simulink model "CtrlCmdCalc"  (R2022b)
settings: Solver=FixedStepDiscrete  StartTime=0.0  StopTime=10.0  FixedStep=0.0001  RelTol=1e-3
values from neighbouring files (symbols this model uses):
  Trq_coeff_Arr_Back_60V = 0.0    [MCU_CtrlCmd.sldd]    (also in MCU_CtrlCmd_objects.m = myPackage.Parameter)
  Trq_coeff_Arr_Back_72V = 0.0    [MCU_CtrlCmd.sldd]    (also in MCU_CtrlCmd_objects.m = myPackage.Parameter)
  Trq_coeff_Arr_HSP_60V = 0.0    [MCU_CtrlCmd.sldd]    (also in MCU_CtrlCmd_objects.m = myPackage.Parameter)
  Trq_coeff_Arr_HSP_72V = 0.0    [MCU_CtrlCmd.sldd]    (also in MCU_CtrlCmd_objects.m = myPackage.Parameter)
  TWISTGRIP_HIGH = 3.3    [MCU_CtrlCmd.sldd]
undefined symbols (not defined in the file or in its folder): ANALOG, cNoneMode, cSpeedLoopMode, cTorqueLoopMode, GEAR, MOTORDIR, ParamCfg_CommandSource_u16, ParamCfg_MaxTorque_u16, POWER_ON, PTIME, STANDBY, TWISTGRIP_UP, TWISTGRIP_VTH_HIGH, TWISTGRIP_VTH_UP
libraries: simulink x2
(part 1 of 2)
settings Model: DataDictionary=MCU_CtrlCmd.sldd  Creator=ZYH  LastModifiedBy=ZYH
settings OptimizationCC: DefaultParameterBehavior=Inlined  EnhancedBackFolding=on  PassReuseOutputArgsAs=Individual arguments  ZeroExternalMemoryAtStartup=off  ZeroInternalMemoryAtStartup=off  OptimizeBlockOrder=speed  DifferentSizesBufferReuse=on  OptimizationCustomize=off  EfficientTunableParamExpr=on
settings DebuggingCC: ParameterTunabilityLossMsg=error
settings SFSimCC: MATLABDynamicMemAlloc=off
settings RTWCC: Description=Embedded Coder  SystemTargetFile=ert.tlc  GenCodeOnly=on  TemplateMakefile=ert_default_tmf
settings CodeAppCC: ForceParamTrailComments=on  IgnoreCustomStorageClasses=off  OperatorAnnotations=on  SimulinkDataObjDesc=on  SFDataObjDesc=on  InsertBlockDesc=on
settings ERTTargetCC: TargetLangStandard=C99 (ISO)  GenerateSampleERTMain=on  InlinedParameterPlacement=NonHierarchical  ERTCustomFileTemplate=example_file_process.tlc

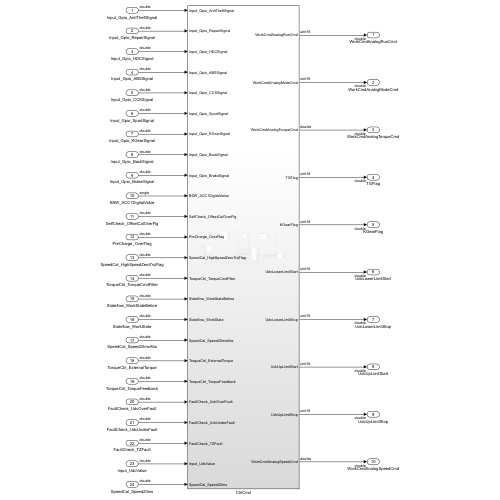
[thumbnail: Simulink's stored preview of the top-level diagram]
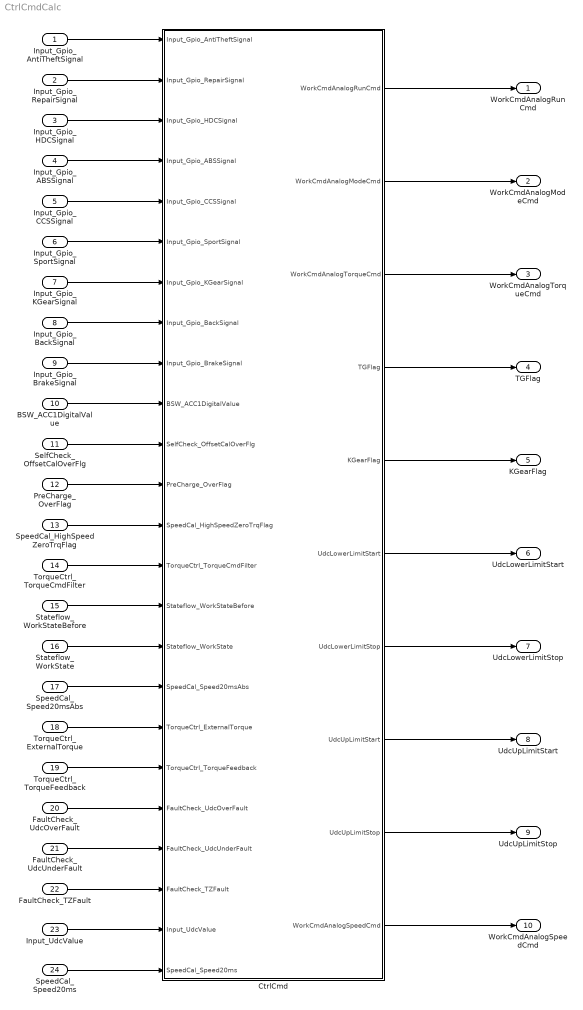
== system CtrlCmdCalc ==
  Input_Gpio_AntiTheftSignal : Inport
  Input_Gpio_RepairSignal : Inport  Port=2
  Input_Gpio_HDCSignal : Inport  Port=3
  Input_Gpio_ABSSignal : Inport  Port=4
  Input_Gpio_CCSSignal : Inport  Port=5
  Input_Gpio_SportSignal : Inport  Port=6
  Input_Gpio_KGearSignal : Inport  Port=7
  Input_Gpio_BackSignal : Inport  Port=8
  Input_Gpio_BrakeSignal : Inport  Port=9
  BSW_ACC1DigitalValue : Inport  Port=10
  SelfCheck_OffsetCalOverFlg : Inport  Port=11
  PreCharge_OverFlag : Inport  Port=12
  SpeedCal_HighSpeedZeroTrqFlag : Inport  Port=13
  TorqueCtrl_TorqueCmdFilter : Inport  Port=14
  Stateflow_WorkStateBefore : Inport  Port=15
  Stateflow_WorkState : Inport  Port=16
  SpeedCal_Speed20msAbs : Inport  Port=17
  TorqueCtrl_ExternalTorque : Inport  Port=18
  TorqueCtrl_TorqueFeedback : Inport  Port=19
  FaultCheck_UdcOverFault : Inport  Port=20
  FaultCheck_UdcUnderFault : Inport  Port=21
  FaultCheck_TZFault : Inport  Port=22
  Input_UdcValue : Inport  Port=23
  SpeedCal_Speed20ms : Inport  Port=24
  CtrlCmd : Subsystem
  WorkCmdAnalogRunCmd : Outport
  WorkCmdAnalogModeCmd : Outport  Port=2
  WorkCmdAnalogTorqueCmd : Outport  Port=3
  TGFlag : Outport  Port=4
  KGearFlag : Outport  Port=5
  UdcLowerLimitStart : Outport  Port=6
  UdcLowerLimitStop : Outport  Port=7
  UdcUpLimitStart : Outport  Port=8
  UdcUpLimitStop : Outport  Port=9
  WorkCmdAnalogSpeedCmd : Outport  Port=10
  wires:
  Input_Gpio_AntiTheftSignal/1 -> CtrlCmd/1(Input_Gpio_AntiTheftSignal)
  Input_Gpio_RepairSignal/1 -> CtrlCmd/2(Input_Gpio_RepairSignal)
  Input_Gpio_HDCSignal/1 -> CtrlCmd/3(Input_Gpio_HDCSignal)
  Input_Gpio_ABSSignal/1 -> CtrlCmd/4(Input_Gpio_ABSSignal)
  Input_Gpio_CCSSignal/1 -> CtrlCmd/5(Input_Gpio_CCSSignal)
  Input_Gpio_SportSignal/1 -> CtrlCmd/6(Input_Gpio_SportSignal)
  Input_Gpio_KGearSignal/1 -> CtrlCmd/7(Input_Gpio_KGearSignal)
  Input_Gpio_BackSignal/1 -> CtrlCmd/8(Input_Gpio_BackSignal)
  Input_Gpio_BrakeSignal/1 -> CtrlCmd/9(Input_Gpio_BrakeSignal)
  BSW_ACC1DigitalValue/1 -> CtrlCmd/10(BSW_ACC1DigitalValue)
  SelfCheck_OffsetCalOverFlg/1 -> CtrlCmd/11(SelfCheck_OffsetCalOverFlg)
  PreCharge_OverFlag/1 -> CtrlCmd/12(PreCharge_OverFlag)
  SpeedCal_HighSpeedZeroTrqFlag/1 -> CtrlCmd/13(SpeedCal_HighSpeedZeroTrqFlag)
  TorqueCtrl_TorqueCmdFilter/1 -> CtrlCmd/14(TorqueCtrl_TorqueCmdFilter)
  Stateflow_WorkStateBefore/1 -> CtrlCmd/15(Stateflow_WorkStateBefore)
  Stateflow_WorkState/1 -> CtrlCmd/16(Stateflow_WorkState)
  SpeedCal_Speed20msAbs/1 -> CtrlCmd/17(SpeedCal_Speed20msAbs)
  TorqueCtrl_ExternalTorque/1 -> CtrlCmd/18(TorqueCtrl_ExternalTorque)
  TorqueCtrl_TorqueFeedback/1 -> CtrlCmd/19(TorqueCtrl_TorqueFeedback)
  FaultCheck_UdcOverFault/1 -> CtrlCmd/20(FaultCheck_UdcOverFault)
  FaultCheck_UdcUnderFault/1 -> CtrlCmd/21(FaultCheck_UdcUnderFault)
  FaultCheck_TZFault/1 -> CtrlCmd/22(FaultCheck_TZFault)
  Input_UdcValue/1 -> CtrlCmd/23(Input_UdcValue)
  SpeedCal_Speed20ms/1 -> CtrlCmd/24(SpeedCal_Speed20ms)
  CtrlCmd/1(WorkCmdAnalogRunCmd) -> WorkCmdAnalogRunCmd/1
  CtrlCmd/2(WorkCmdAnalogModeCmd) -> WorkCmdAnalogModeCmd/1
  CtrlCmd/3(WorkCmdAnalogTorqueCmd) -> WorkCmdAnalogTorqueCmd/1
  CtrlCmd/4(TGFlag) -> TGFlag/1
  CtrlCmd/5(KGearFlag) -> KGearFlag/1
  CtrlCmd/6(UdcLowerLimitStart) -> UdcLowerLimitStart/1
  CtrlCmd/7(UdcLowerLimitStop) -> UdcLowerLimitStop/1
  CtrlCmd/8(UdcUpLimitStart) -> UdcUpLimitStart/1
  CtrlCmd/9(UdcUpLimitStop) -> UdcUpLimitStop/1
  CtrlCmd/10(WorkCmdAnalogSpeedCmd) -> WorkCmdAnalogSpeedCmd/1

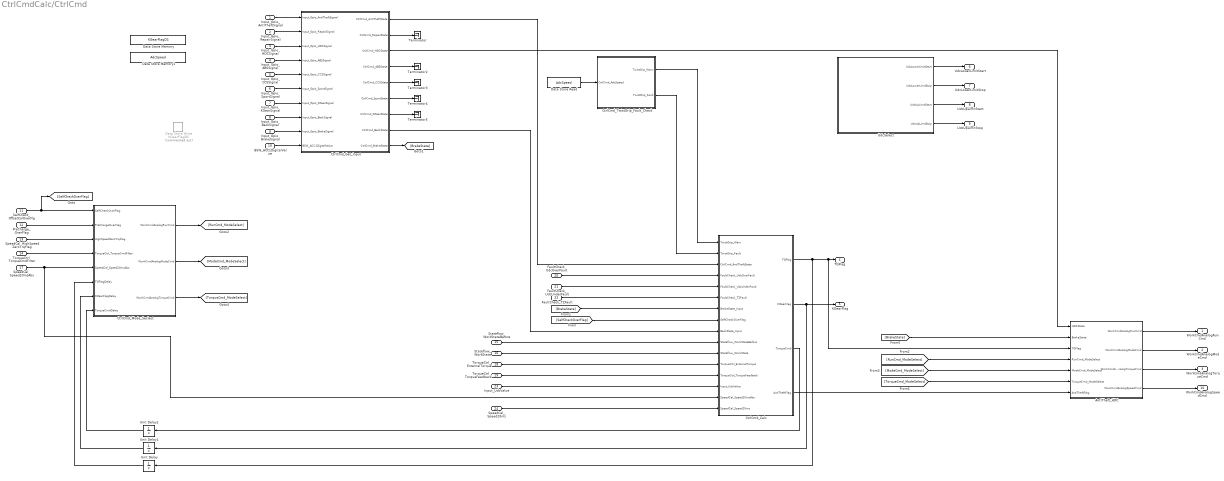
== system CtrlCmdCalc/CtrlCmd ==
  Input_Gpio_AntiTheftSignal : Inport
  Input_Gpio_RepairSignal : Inport  Port=2
  Input_Gpio_HDCSignal : Inport  Port=3
  Input_Gpio_ABSSignal : Inport  Port=4
  Input_Gpio_CCSSignal : Inport  Port=5
  Input_Gpio_SportSignal : Inport  Port=6
  Input_Gpio_KGearSignal : Inport  Port=7
  Input_Gpio_BackSignal : Inport  Port=8
  Input_Gpio_BrakeSignal : Inport  Port=9
  BSW_ACC1DigitalValue : Inport  Port=10
  SelfCheck_OffsetCalOverFlg : Inport  Port=11
  PreCharge_OverFlag : Inport  Port=12
  SpeedCal_HighSpeedZeroTrqFlag : Inport  Port=13
  TorqueCtrl_TorqueCmdFilter : Inport  Port=14
  Stateflow_WorkStateBefore : Inport  Port=15
  Stateflow_WorkState : Inport  Port=16
  SpeedCal_Speed20msAbs : Inport  Port=17
  TorqueCtrl_ExternalTorque : Inport  Port=18
  TorqueCtrl_TorqueFeedback : Inport  Port=19
  FaultCheck_UdcOverFault : Inport  Port=20
  FaultCheck_UdcUnderFault : Inport  Port=21
  FaultCheck_TZFault : Inport  Port=22
  Input_UdcValue : Inport  Port=23
  SpeedCal_Speed20ms : Inport  Port=24
  AntiTheft_HDC : Subsystem
  CtrlCmd_Calc : Subsystem
  CtrlCmd_Get_Input : Subsystem
  CtrlCmd_Mode_Seclect : Subsystem
  CtrlCmd_TwistGrip_Fault_Check : Subsystem
  Data Store Memory : DataStoreMemory  DataStoreName=KGearFlagDS  WriteAfterWriteMsg=warning  InitialValue=3  ShowAdditionalParam=off  OutDataTypeStr=uint16
  Data Store Memory1 : DataStoreMemory  DataStoreName=AdcSpeed  WriteAfterWriteMsg=warning  ShowAdditionalParam=off  OutDataTypeStr=single
  Data Store Read : DataStoreRead  DataStoreName=AdcSpeed  IndexOptions=Index vector (dialog)  Indices=1  OutputSizes=1
  Data Store Write : DataStoreWrite  Commented=on  DataStoreName=KGearFlagDS  IndexOptions=Index vector (dialog)  Indices=1  OutputSizes=1
  Terminator{,2..5} (5 alike) : Terminator
  UdcSelect : Subsystem
  Unit Delay : UnitDelay  SampleTime=-1  HasFrameUpgradeWarning=on
  Unit Delay1 : UnitDelay  SampleTime=-1  HasFrameUpgradeWarning=on
  Unit Delay2 : UnitDelay  SampleTime=-1  HasFrameUpgradeWarning=on
  WorkCmdAnalogRunCmd : Outport
  WorkCmdAnalogModeCmd : Outport  Port=2
  WorkCmdAnalogTorqueCmd : Outport  Port=3
  TGFlag : Outport  Port=4
  KGearFlag : Outport  Port=5
  UdcLowerLimitStart : Outport  Port=6
  UdcLowerLimitStop : Outport  Port=7
  UdcUpLimitStart : Outport  Port=8
  UdcUpLimitStop : Outport  Port=9
  WorkCmdAnalogSpeedCmd : Outport  Port=10
  wires:
  Input_Gpio_AntiTheftSignal/1 -> CtrlCmd_Get_Input/1(Input_Gpio_AntiTheftSignal)
  Input_Gpio_RepairSignal/1 -> CtrlCmd_Get_Input/2(Input_Gpio_RepairSignal)
  Input_Gpio_HDCSignal/1 -> CtrlCmd_Get_Input/3(Input_Gpio_HDCSignal)
  Input_Gpio_ABSSignal/1 -> CtrlCmd_Get_Input/4(Input_Gpio_ABSSignal)
  Input_Gpio_CCSSignal/1 -> CtrlCmd_Get_Input/5(Input_Gpio_CCSSignal)
  Input_Gpio_SportSignal/1 -> CtrlCmd_Get_Input/6(Input_Gpio_SportSignal)
  Input_Gpio_KGearSignal/1 -> CtrlCmd_Get_Input/7(Input_Gpio_KGearSignal)
  Input_Gpio_BackSignal/1 -> CtrlCmd_Get_Input/8(Input_Gpio_BackSignal)
  Input_Gpio_BrakeSignal/1 -> CtrlCmd_Get_Input/9(Input_Gpio_BrakeSignal)
  BSW_ACC1DigitalValue/1 -> CtrlCmd_Get_Input/10(BSW_ACC1DigitalValue)
  SelfCheck_OffsetCalOverFlg/1 -> [SelfCheckOverFlag], CtrlCmd_Mode_Seclect/1(SelfCheckOverFlag)
  Data Store Read/1 -> CtrlCmd_TwistGrip_Fault_Check/1(CtrlCmd_AdcSpeed)
  PreCharge_OverFlag/1 -> CtrlCmd_Mode_Seclect/2(PreChargeOverFlag)
  SpeedCal_HighSpeedZeroTrqFlag/1 -> CtrlCmd_Mode_Seclect/3(HighSpeedZeroTrqFlag)
  TorqueCtrl_TorqueCmdFilter/1 -> CtrlCmd_Mode_Seclect/4(TorqueCtrl_TorqueCmdFilter)
  CtrlCmd_Calc/1(TGFlag) -> AntiTheft_HDC/3(TGFlag), TGFlag/1, Unit Delay/1
  Unit Delay/1 -> CtrlCmd_Mode_Seclect/6(TGFlagDelay)
  CtrlCmd_Calc/2(KGearFlag) -> KGearFlag/1, Unit Delay1/1
  Unit Delay1/1 -> CtrlCmd_Mode_Seclect/7(KGearFlagDelay)
  CtrlCmd_Calc/3(TorqueCmd) -> Unit Delay2/1
  Unit Delay2/1 -> CtrlCmd_Mode_Seclect/8(TorqueCmdDelay)
  SpeedCal_Speed20msAbs/1 -> CtrlCmd_Mode_Seclect/5(SpeedCal_Speed20msAbs), CtrlCmd_Calc/15(SpeedCal_Speed20msAbs)
  Stateflow_WorkStateBefore/1 -> CtrlCmd_Calc/10(Stateflow_WorkStateBefore)
  Stateflow_WorkState/1 -> CtrlCmd_Calc/11(Stateflow_WorkState)
  TorqueCtrl_ExternalTorque/1 -> CtrlCmd_Calc/12(TorqueCtrl_ExternalTorque)
  TorqueCtrl_TorqueFeedback/1 -> CtrlCmd_Calc/13(TorqueCtrl_TorqueFeedback)
  [SelfCheckOverFlag] -> CtrlCmd_Calc/8(SelfCheckOverFlag)
  CtrlCmd_Get_Input/9(CtrlCmd_BrakeState) -> [BrakeState]
  [BrakeState] -> CtrlCmd_Calc/7(BrakeState_Input)
  CtrlCmd_Get_Input/1(CtrlCmd_AntiTheftState) -> CtrlCmd_Calc/3(CtrlCmd_AntiTheftState)
  FaultCheck_TZFault/1 -> CtrlCmd_Calc/6(FaultCheck_TZFault)
  FaultCheck_UdcOverFault/1 -> CtrlCmd_Calc/4(FaultCheck_UdcOverFault)
  FaultCheck_UdcUnderFault/1 -> CtrlCmd_Calc/5(FaultCheck_UdcUnderFault)
  CtrlCmd_TwistGrip_Fault_Check/1(TwistGrip_Warn) -> CtrlCmd_Calc/1(TwistGrip_Warn)
  CtrlCmd_TwistGrip_Fault_Check/2(TwistGrip_Fault) -> CtrlCmd_Calc/2(TwistGrip_Fault)
  CtrlCmd_Get_Input/8(CtrlCmd_BackState) -> CtrlCmd_Calc/9(BackState_Input)
  Input_UdcValue/1 -> CtrlCmd_Calc/14(Input_UdcValue)
  SpeedCal_Speed20ms/1 -> CtrlCmd_Calc/16(SpeedCal_Speed20ms)
  CtrlCmd_Get_Input/2(CtrlCmd_RepairState) -> Terminator/1
  CtrlCmd_Get_Input/4(CtrlCmd_ABSState) -> Terminator2/1
  CtrlCmd_Get_Input/5(CtrlCmd_CCSState) -> Terminator3/1
  CtrlCmd_Get_Input/6(CtrlCmd_SportState) -> Terminator4/1
  CtrlCmd_Get_Input/7(CtrlCmd_KGearState) -> Terminator5/1
  UdcSelect/1(UdcLowerLimitStart) -> UdcLowerLimitStart/1
  UdcSelect/2(UdcLowerLimitStop) -> UdcLowerLimitStop/1
  UdcSelect/3(UdcUpLimitStart) -> UdcUpLimitStart/1
  UdcSelect/4(UdcUpLimitStop) -> UdcUpLimitStop/1
  CtrlCmd_Calc/4(AntiTheftFlag) -> AntiTheft_HDC/7(AntiTheftFlag)
  CtrlCmd_Mode_Seclect/3(WorkCmdAnalogTorqueCmd) -> [TorqueCmd_ModeSelect]
  CtrlCmd_Mode_Seclect/2(WorkCmdAnalogModeCmd) -> [ModeCmd_ModeSelect]
  CtrlCmd_Mode_Seclect/1(WorkCmdAnalogRunCmd) -> [RunCmd_ModeSelect]
  [TorqueCmd_ModeSelect] -> AntiTheft_HDC/6(TorqueCmd_ModeSelect)
  [ModeCmd_ModeSelect] -> AntiTheft_HDC/5(ModeCmd_ModeSelect)
  [RunCmd_ModeSelect] -> AntiTheft_HDC/4(RunCmd_ModeSelect)
  CtrlCmd_Get_Input/3(CtrlCmd_HDCState) -> AntiTheft_HDC/1(HDCState)
  [BrakeState] -> AntiTheft_HDC/2(BrakeState)
  AntiTheft_HDC/1(WorkCmdAnalogRunCmd) -> WorkCmdAnalogRunCmd/1
  AntiTheft_HDC/2(WorkCmdAnalogModeCmd) -> WorkCmdAnalogModeCmd/1
  AntiTheft_HDC/3(WorkCmdAnalogTorqueCmd) -> WorkCmdAnalogTorqueCmd/1
  AntiTheft_HDC/4(WorkCmdAnalogSpeedCmd) -> WorkCmdAnalogSpeedCmd/1

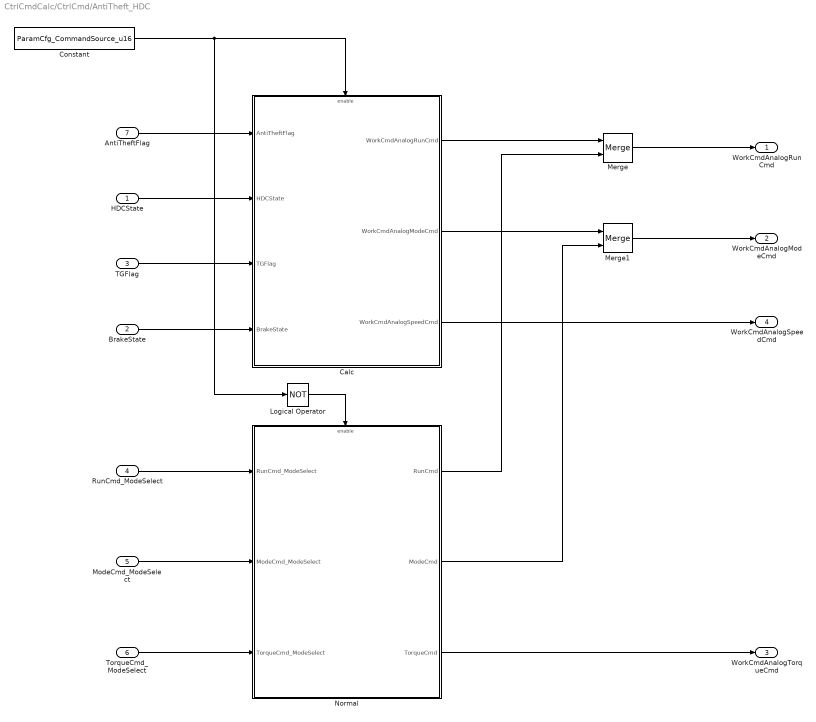
== system CtrlCmdCalc/CtrlCmd/AntiTheft_HDC ==
  HDCState : Inport
  BrakeState : Inport  Port=2
  TGFlag : Inport  Port=3
  RunCmd_ModeSelect : Inport  Port=4
  ModeCmd_ModeSelect : Inport  Port=5
  TorqueCmd_ModeSelect : Inport  Port=6
  AntiTheftFlag : Inport  Port=7
  Calc : Subsystem  TreatAsAtomicUnit=on
  Constant : Constant  Value=ParamCfg_CommandSource_u16
  Logical Operator : Logic  Operator=NOT  AllPortsSameDT=off  OutDataTypeStr=boolean
  Merge : Merge
  Merge1 : Merge
  Normal : Subsystem
  WorkCmdAnalogRunCmd : Outport
  WorkCmdAnalogModeCmd : Outport  Port=2
  WorkCmdAnalogTorqueCmd : Outport  Port=3
  WorkCmdAnalogSpeedCmd : Outport  Port=4
  wires:
  Constant/1 -> Logical Operator/1, Calc/Enable
  AntiTheftFlag/1 -> Calc/1(AntiTheftFlag)
  RunCmd_ModeSelect/1 -> Normal/1(RunCmd_ModeSelect)
  ModeCmd_ModeSelect/1 -> Normal/2(ModeCmd_ModeSelect)
  TorqueCmd_ModeSelect/1 -> Normal/3(TorqueCmd_ModeSelect)
  Logical Operator/1 -> Normal/Enable
  Calc/1(WorkCmdAnalogRunCmd) -> Merge/1
  Merge/1 -> WorkCmdAnalogRunCmd/1
  Calc/2(WorkCmdAnalogModeCmd) -> Merge1/1
  Normal/1(RunCmd) -> Merge/2
  Normal/2(ModeCmd) -> Merge1/2
  Merge1/1 -> WorkCmdAnalogModeCmd/1
  HDCState/1 -> Calc/2(HDCState)
  TGFlag/1 -> Calc/3(TGFlag)
  BrakeState/1 -> Calc/4(BrakeState)
  Calc/3(WorkCmdAnalogSpeedCmd) -> WorkCmdAnalogSpeedCmd/1
  Normal/3(TorqueCmd) -> WorkCmdAnalogTorqueCmd/1

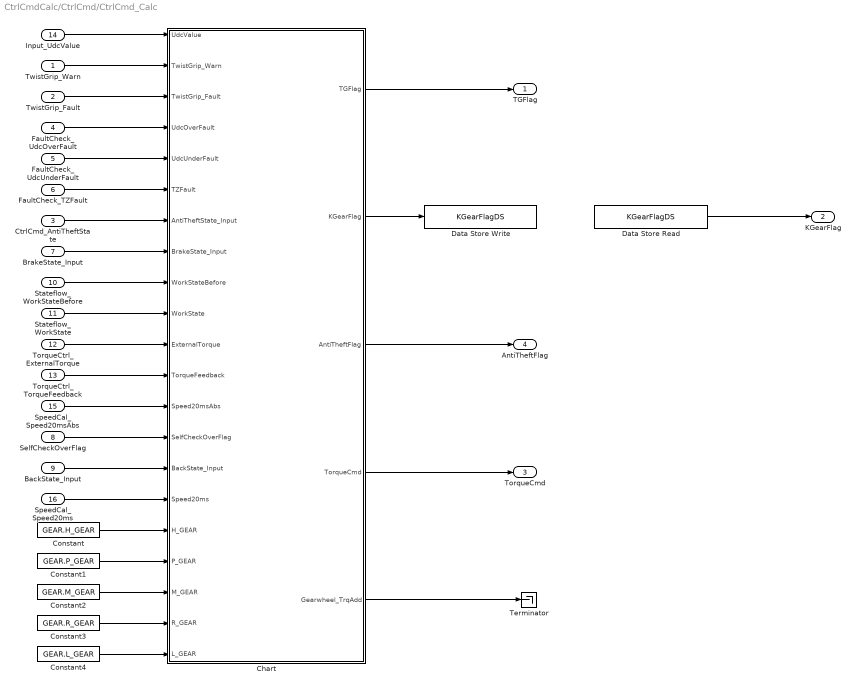
== system CtrlCmdCalc/CtrlCmd/CtrlCmd_Calc ==
  TwistGrip_Warn : Inport
  TwistGrip_Fault : Inport  Port=2
  CtrlCmd_AntiTheftState : Inport  Port=3
  FaultCheck_UdcOverFault : Inport  Port=4
  FaultCheck_UdcUnderFault : Inport  Port=5
  FaultCheck_TZFault : Inport  Port=6
  BrakeState_Input : Inport  Port=7
  SelfCheckOverFlag : Inport  Port=8
  BackState_Input : Inport  Port=9
  Stateflow_WorkStateBefore : Inport  Port=10
  Stateflow_WorkState : Inport  Port=11
  TorqueCtrl_ExternalTorque : Inport  Port=12
  TorqueCtrl_TorqueFeedback : Inport  Port=13
  Input_UdcValue : Inport  Port=14
  SpeedCal_Speed20msAbs : Inport  Port=15
  SpeedCal_Speed20ms : Inport  Port=16
  Chart : Stateflow chart  TreatAsAtomicUnit=on
      settings: PortSchema="{\"entries\":[{\"content\":{\"sides\":[{\"content\":{\"connectorIds\":[\"In1\",\"In3\",\"In2\",\"In5\",\"In4\",\"In6\",\"In7\",\"In8\",\"In9\",\"In10\",\"In11\",\"In12\",\"In13\",\"In15\",\"In20\",\"In21\",\"In14\",\"In16\",\"In17\",\"In18\",\"In19\"]},\"type\":\"ConnectorPlacement.EquallySpacedRectSide\",\"uuid\":\"3ac4e098-dcda-4c80-8391-2c23d040ea90\"},{\"content\":{\"connectorIds\":[\"Out1\",\"Out2\",\"Out3\",\"Out4\",\"Out5\"],\"side\":\"RIGHT\"},\"type\":\"ConnectorPlacement.EquallySpacedRectSide\",\"uuid\":\"2a9563d8-bf95-4ba8-8718-9ed08349656d\"},{\"content\":{\"connectorIds\":[],\"side\":\"TOP\"},\"type\":\"ConnectorPlacement.EquallySpacedRectSide\",\"uuid\":\"a1bb8453-bbab-459c-b3f0-24bc29724271\"}]},\"type\":\"ConnectorPlacement.EquallySpacedConnector\",\"uuid\":\"5f95f66f-474b-4a0c-911a-4da2c08bb750\"}],\"packageUris\":[\"http://schema.mathworks.com/mf0/Connector/R2020b\"],\"version\":\"1.0\"}"
  Constant : Constant  Value=GEAR.H_GEAR
  Constant1 : Constant  Value=GEAR.P_GEAR
  Constant2 : Constant  Value=GEAR.M_GEAR
  Constant3 : Constant  Value=GEAR.R_GEAR
  Constant4 : Constant  Value=GEAR.L_GEAR
  Data Store Read : DataStoreRead  DataStoreName=KGearFlagDS  IndexOptions=Index vector (dialog)  Indices=1  OutputSizes=1
  Data Store Write : DataStoreWrite  DataStoreName=KGearFlagDS  IndexOptions=Index vector (dialog)  Indices=1  OutputSizes=1
  Terminator : Terminator
  TGFlag : Outport
  KGearFlag : Outport  Port=2
  TorqueCmd : Outport  Port=3
  AntiTheftFlag : Outport  Port=4
  wires:
  Stateflow_WorkStateBefore/1 -> Chart/9(WorkStateBefore)
  Stateflow_WorkState/1 -> Chart/10(WorkState)
  TorqueCtrl_ExternalTorque/1 -> Chart/11(ExternalTorque)
  TorqueCtrl_TorqueFeedback/1 -> Chart/12(TorqueFeedback)
  SpeedCal_Speed20msAbs/1 -> Chart/13(Speed20msAbs)
  Chart/2(KGearFlag) -> Data Store Write/1
  Constant/1 -> Chart/14(H_GEAR)
  SelfCheckOverFlag/1 -> Chart/15(SelfCheckOverFlag)
  Constant1/1 -> Chart/16(P_GEAR)
  BrakeState_Input/1 -> Chart/8(BrakeState_Input)
  Constant2/1 -> Chart/17(M_GEAR)
  Data Store Read/1 -> KGearFlag/1
  Chart/1(TGFlag) -> TGFlag/1
  Constant3/1 -> Chart/18(R_GEAR)
  CtrlCmd_AntiTheftState/1 -> Chart/7(AntiTheftState_Input)
  Chart/3(AntiTheftFlag) -> AntiTheftFlag/1
  TwistGrip_Warn/1 -> Chart/3(TwistGrip_Warn)
  TwistGrip_Fault/1 -> Chart/2(TwistGrip_Fault)
  FaultCheck_UdcOverFault/1 -> Chart/5(UdcOverFault)
  FaultCheck_UdcUnderFault/1 -> Chart/4(UdcUnderFault)
  FaultCheck_TZFault/1 -> Chart/6(TZFault)
  Constant4/1 -> Chart/19(L_GEAR)
  BackState_Input/1 -> Chart/20(BackState_Input)
  Chart/4(TorqueCmd) -> TorqueCmd/1
  Input_UdcValue/1 -> Chart/1(UdcValue)
  Chart/5(Gearwheel_TrqAdd) -> Terminator/1
  SpeedCal_Speed20ms/1 -> Chart/21(Speed20ms)

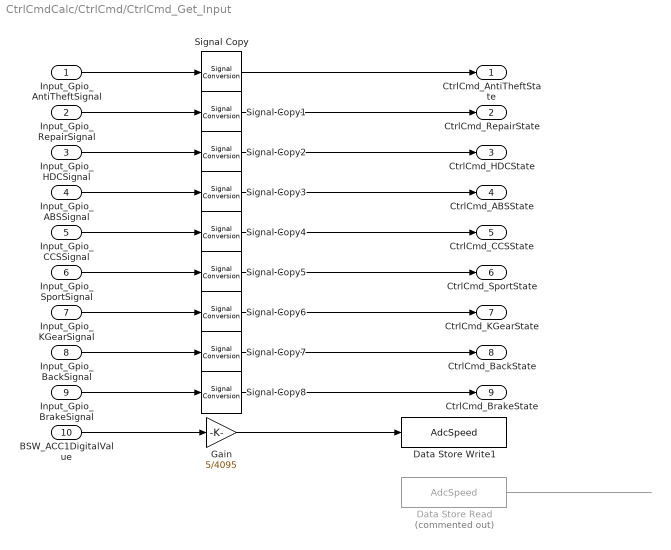
== system CtrlCmdCalc/CtrlCmd/CtrlCmd_Get_Input ==
  Input_Gpio_AntiTheftSignal : Inport
  Input_Gpio_RepairSignal : Inport  Port=2
  Input_Gpio_HDCSignal : Inport  Port=3
  Input_Gpio_ABSSignal : Inport  Port=4
  Input_Gpio_CCSSignal : Inport  Port=5
  Input_Gpio_SportSignal : Inport  Port=6
  Input_Gpio_KGearSignal : Inport  Port=7
  Input_Gpio_BackSignal : Inport  Port=8
  Input_Gpio_BrakeSignal : Inport  Port=9
  BSW_ACC1DigitalValue : Inport  Port=10
  Data Store Read : DataStoreRead  Commented=on  DataStoreName=AdcSpeed  IndexOptions=Index vector (dialog)  Indices=1  OutputSizes=1
  Data Store Write1 : DataStoreWrite  DataStoreName=AdcSpeed  IndexOptions=Index vector (dialog)  Indices=1  OutputSizes=1
  Gain : Gain  Gain=5/4095  ParamDataTypeStr=single  OutDataTypeStr=single
      settings: AttributesFormatString=%<Gain>
  Signal Copy{,1..8} (9 alike) : SignalConversion  OverrideOpt=off
  CtrlCmd_AntiTheftState : Outport
  CtrlCmd_RepairState : Outport  Port=2
  CtrlCmd_HDCState : Outport  Port=3
  CtrlCmd_ABSState : Outport  Port=4
  CtrlCmd_CCSState : Outport  Port=5
  CtrlCmd_SportState : Outport  Port=6
  CtrlCmd_KGearState : Outport  Port=7
  CtrlCmd_BackState : Outport  Port=8
  CtrlCmd_BrakeState : Outport  Port=9
  wires:
  Input_Gpio_AntiTheftSignal/1 -> Signal Copy/1
  Input_Gpio_RepairSignal/1 -> Signal Copy1/1
  Input_Gpio_HDCSignal/1 -> Signal Copy2/1
  Input_Gpio_ABSSignal/1 -> Signal Copy3/1
  Input_Gpio_CCSSignal/1 -> Signal Copy4/1
  Input_Gpio_SportSignal/1 -> Signal Copy5/1
  Input_Gpio_KGearSignal/1 -> Signal Copy6/1
  Input_Gpio_BackSignal/1 -> Signal Copy7/1
  Input_Gpio_BrakeSignal/1 -> Signal Copy8/1
  BSW_ACC1DigitalValue/1 -> Gain/1
  Gain/1 -> Data Store Write1/1
  Signal Copy/1 -> CtrlCmd_AntiTheftState/1
  Signal Copy1/1 -> CtrlCmd_RepairState/1
  Signal Copy8/1 -> CtrlCmd_BrakeState/1
  Signal Copy7/1 -> CtrlCmd_BackState/1
  Signal Copy6/1 -> CtrlCmd_KGearState/1
  Signal Copy5/1 -> CtrlCmd_SportState/1
  Signal Copy4/1 -> CtrlCmd_CCSState/1
  Signal Copy3/1 -> CtrlCmd_ABSState/1
  Signal Copy2/1 -> CtrlCmd_HDCState/1
  Data Store Read/1 -> ?

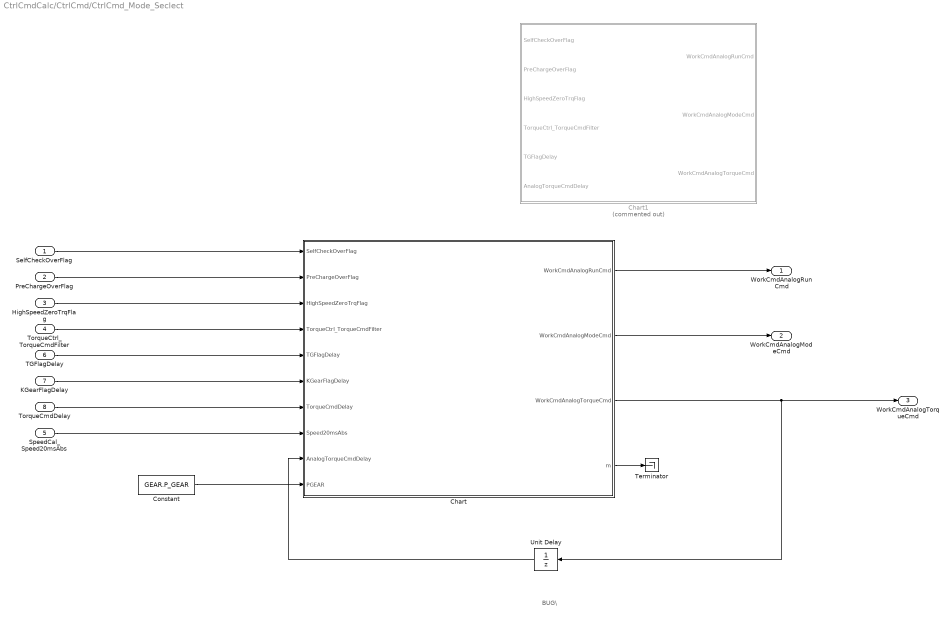
== system CtrlCmdCalc/CtrlCmd/CtrlCmd_Mode_Seclect ==
  note: BUG\
  SelfCheckOverFlag : Inport
  PreChargeOverFlag : Inport  Port=2
  HighSpeedZeroTrqFlag : Inport  Port=3
  TorqueCtrl_TorqueCmdFilter : Inport  Port=4
  SpeedCal_Speed20msAbs : Inport  Port=5
  TGFlagDelay : Inport  Port=6
  KGearFlagDelay : Inport  Port=7
  TorqueCmdDelay : Inport  Port=8
  Chart : Stateflow chart  TreatAsAtomicUnit=on
      settings: PortSchema="{\"entries\":[{\"content\":{\"sides\":[{\"content\":{\"connectorIds\":[\"In1\",\"In2\",\"In3\",\"In4\",\"In5\",\"In9\",\"In7\",\"In8\",\"In6\",\"In10\"]},\"type\":\"ConnectorPlacement.EquallySpacedRectSide\",\"uuid\":\"b2d776f0-2615-48a9-a6c0-c843049782f9\"},{\"content\":{\"connectorIds\":[\"Out1\",\"Out2\",\"Out3\",\"Out4\"],\"side\":\"RIGHT\"},\"type\":\"ConnectorPlacement.EquallySpacedRectSide\",\"uuid\":\"8bd2f04f-8b65-482d-924a-cc36ec8f1c20\"},{\"content\":{\"connectorIds\":[],\"side\":\"TOP\"},\"type\":\"ConnectorPlacement.EquallySpacedRectSide\",\"uuid\":\"4fb49ddf-20a5-44b1-930a-29191850c309\"}]},\"type\":\"ConnectorPlacement.EquallySpacedConnector\",\"uuid\":\"dc35ac27-112e-45e7-b1c8-84497b20d01d\"}],\"packageUris\":[\"http://schema.mathworks.com/mf0/Connector/R2020b\"],\"version\":\"1.0\"}"
  Chart1 : Stateflow chart  Commented=on  TreatAsAtomicUnit=on
  Constant : Constant  Value=GEAR.P_GEAR
  Terminator : Terminator
  Unit Delay : UnitDelay  SampleTime=-1  HasFrameUpgradeWarning=on
  WorkCmdAnalogRunCmd : Outport
  WorkCmdAnalogModeCmd : Outport  Port=2
  WorkCmdAnalogTorqueCmd : Outport  Port=3
  wires:
  SelfCheckOverFlag/1 -> Chart/1(SelfCheckOverFlag)
  PreChargeOverFlag/1 -> Chart/2(PreChargeOverFlag)
  HighSpeedZeroTrqFlag/1 -> Chart/3(HighSpeedZeroTrqFlag)
  TorqueCtrl_TorqueCmdFilter/1 -> Chart/4(TorqueCtrl_TorqueCmdFilter)
  TGFlagDelay/1 -> Chart/5(TGFlagDelay)
  Chart/3(WorkCmdAnalogTorqueCmd) -> Unit Delay/1, WorkCmdAnalogTorqueCmd/1
  Unit Delay/1 -> Chart/6(AnalogTorqueCmdDelay)
  KGearFlagDelay/1 -> Chart/9(KGearFlagDelay)
  Constant/1 -> Chart/10(PGEAR)
  TorqueCmdDelay/1 -> Chart/7(TorqueCmdDelay)
  SpeedCal_Speed20msAbs/1 -> Chart/8(Speed20msAbs)
  Chart/4(m) -> Terminator/1
  Chart/2(WorkCmdAnalogModeCmd) -> WorkCmdAnalogModeCmd/1
  Chart/1(WorkCmdAnalogRunCmd) -> WorkCmdAnalogRunCmd/1

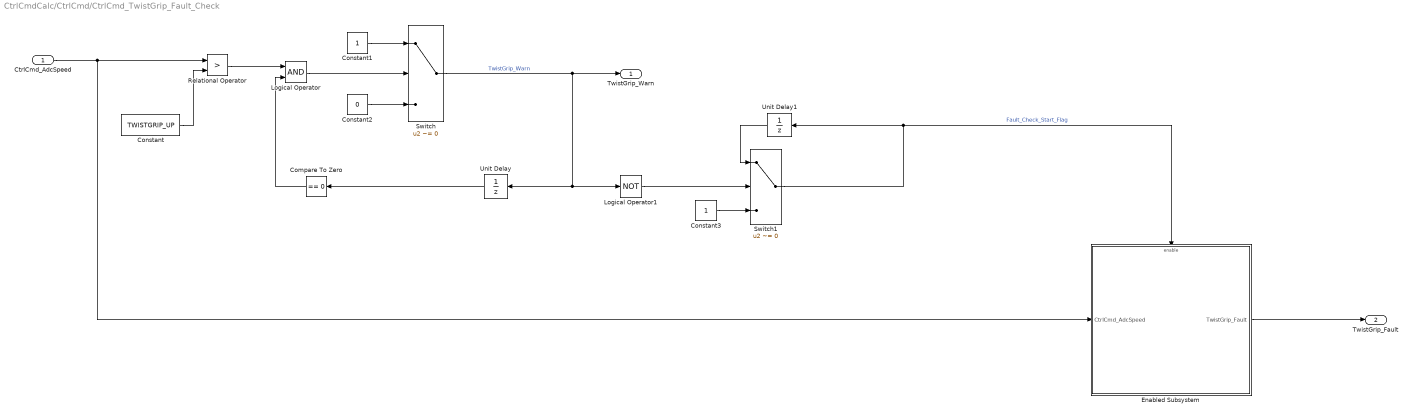
== system CtrlCmdCalc/CtrlCmd/CtrlCmd_TwistGrip_Fault_Check ==
  CtrlCmd_AdcSpeed : Inport
  Compare To Zero : simulink/Logic and Bit Operations/Compare To Zero  relop===  OutDataTypeStr=boolean
  Constant : Constant  Value=TWISTGRIP_UP
  Constant1 : Constant  OutDataTypeStr=uint8
  Constant2 : Constant  Value=0  OutDataTypeStr=uint8
  Constant3 : Constant  OutDataTypeStr=uint8
  Enabled Subsystem : Subsystem  TreatAsAtomicUnit=on
  Logical Operator : Logic  AllPortsSameDT=off  OutDataTypeStr=boolean
  Logical Operator1 : Logic  Operator=NOT  AllPortsSameDT=off  OutDataTypeStr=boolean
  Relational Operator : RelationalOperator  Operator=>  OutDataTypeStr=boolean  RndMeth=Simplest  InputSameDT=off
  Switch : Switch  Criteria=u2 ~= 0  SaturateOnIntegerOverflow=off  InputSameDT=off
  Switch1 : Switch  Criteria=u2 ~= 0  SaturateOnIntegerOverflow=off  InputSameDT=off
  Unit Delay : UnitDelay  SampleTime=-1  HasFrameUpgradeWarning=on
  Unit Delay1 : UnitDelay  SampleTime=-1  HasFrameUpgradeWarning=on
  TwistGrip_Warn : Outport
  TwistGrip_Fault : Outport  Port=2
  wires:
  CtrlCmd_AdcSpeed/1 -> Enabled Subsystem/1(CtrlCmd_AdcSpeed), Relational Operator/1
  Constant/1 -> Relational Operator/2
  Relational Operator/1 -> Logical Operator/1
  Switch/1 -> Unit Delay/1, Logical Operator1/1, TwistGrip_Warn/1  "TwistGrip_Warn"
  Unit Delay/1 -> Compare To Zero/1
  Compare To Zero/1 -> Logical Operator/2
  Logical Operator/1 -> Switch/2
  Constant1/1 -> Switch/1
  Constant2/1 -> Switch/3
  Switch1/1 -> Enabled Subsystem/Enable, Unit Delay1/1  "Fault_Check_Start_Flag"
  Logical Operator1/1 -> Switch1/2
  Constant3/1 -> Switch1/3
  Unit Delay1/1 -> Switch1/1
  Enabled Subsystem/1(TwistGrip_Fault) -> TwistGrip_Fault/1

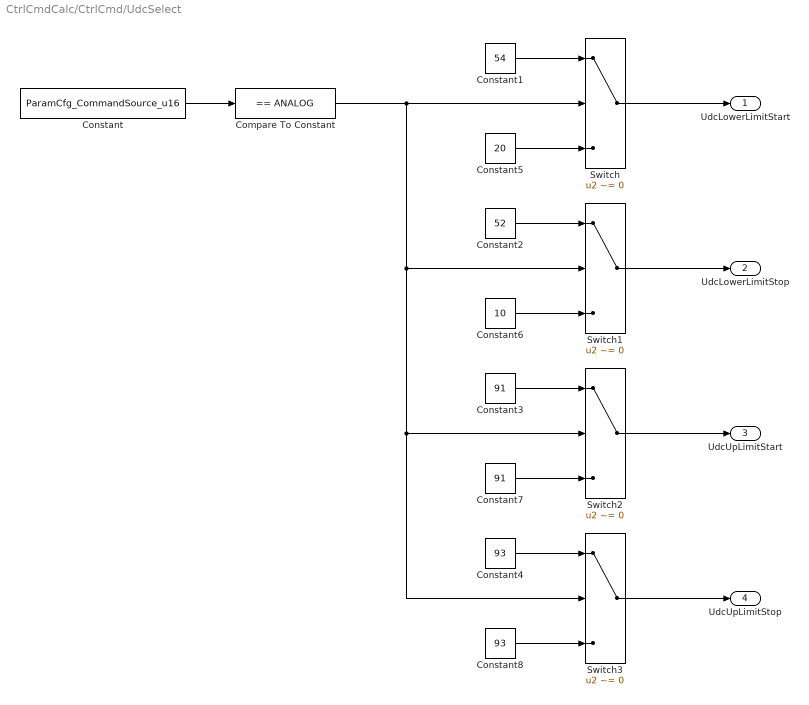
== system CtrlCmdCalc/CtrlCmd/UdcSelect ==
  Compare To Constant : simulink/Logic and Bit Operations/Compare To Constant  relop===  const=ANALOG  OutDataTypeStr=boolean
  Constant : Constant  Value=ParamCfg_CommandSource_u16
  Constant1 : Constant  Value=54  OutDataTypeStr=uint16
  Constant2 : Constant  Value=52  OutDataTypeStr=uint16
  Constant3 : Constant  Value=91  OutDataTypeStr=uint16
  Constant4 : Constant  Value=93  OutDataTypeStr=uint16
  Constant5 : Constant  Value=20  OutDataTypeStr=uint16
  Constant6 : Constant  Value=10  OutDataTypeStr=uint16
  Constant7 : Constant  Value=91  OutDataTypeStr=uint16
  Constant8 : Constant  Value=93  OutDataTypeStr=uint16
  Switch{,1..3} (4 alike) : Switch  Criteria=u2 ~= 0  SaturateOnIntegerOverflow=off  InputSameDT=off
  UdcLowerLimitStart : Outport
  UdcLowerLimitStop : Outport  Port=2
  UdcUpLimitStart : Outport  Port=3
  UdcUpLimitStop : Outport  Port=4
  wires:
  Constant/1 -> Compare To Constant/1
  Compare To Constant/1 -> Switch/2, Switch1/2, Switch2/2, Switch3/2
  Switch/1 -> UdcLowerLimitStart/1
  Switch1/1 -> UdcLowerLimitStop/1
  Switch2/1 -> UdcUpLimitStart/1
  Switch3/1 -> UdcUpLimitStop/1
  Constant1/1 -> Switch/1
  Constant2/1 -> Switch1/1
  Constant3/1 -> Switch2/1
  Constant4/1 -> Switch3/1
  Constant5/1 -> Switch/3
  Constant6/1 -> Switch1/3
  Constant7/1 -> Switch2/3
  Constant8/1 -> Switch3/3

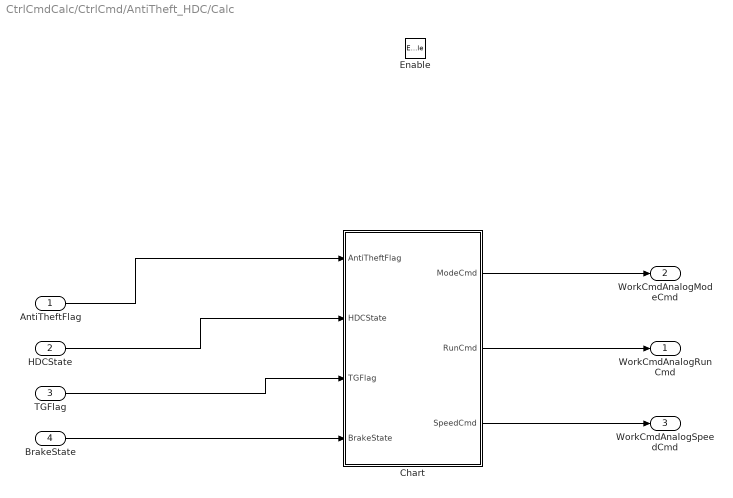
== system CtrlCmdCalc/CtrlCmd/AntiTheft_HDC/Calc ==
  AntiTheftFlag : Inport
  HDCState : Inport  Port=2
  TGFlag : Inport  Port=3
  BrakeState : Inport  Port=4
  Enable : EnablePort
  Chart : Stateflow chart  TreatAsAtomicUnit=on
  WorkCmdAnalogRunCmd : Outport
  WorkCmdAnalogModeCmd : Outport  Port=2
  WorkCmdAnalogSpeedCmd : Outport  Port=3
  wires:
  AntiTheftFlag/1 -> Chart/1(AntiTheftFlag)
  HDCState/1 -> Chart/2(HDCState)
  TGFlag/1 -> Chart/3(TGFlag)
  BrakeState/1 -> Chart/4(BrakeState)
  Chart/1(ModeCmd) -> WorkCmdAnalogModeCmd/1
  Chart/2(RunCmd) -> WorkCmdAnalogRunCmd/1
  Chart/3(SpeedCmd) -> WorkCmdAnalogSpeedCmd/1

== system CtrlCmdCalc/CtrlCmd/AntiTheft_HDC/Normal ==
  RunCmd_ModeSelect : Inport
  ModeCmd_ModeSelect : Inport  Port=2
  TorqueCmd_ModeSelect : Inport  Port=3
  Enable : EnablePort
  RunCmd : Outport
  ModeCmd : Outport  Port=2
  TorqueCmd : Outport  Port=3
  wires:
  RunCmd_ModeSelect/1 -> RunCmd/1
  ModeCmd_ModeSelect/1 -> ModeCmd/1
  TorqueCmd_ModeSelect/1 -> TorqueCmd/1

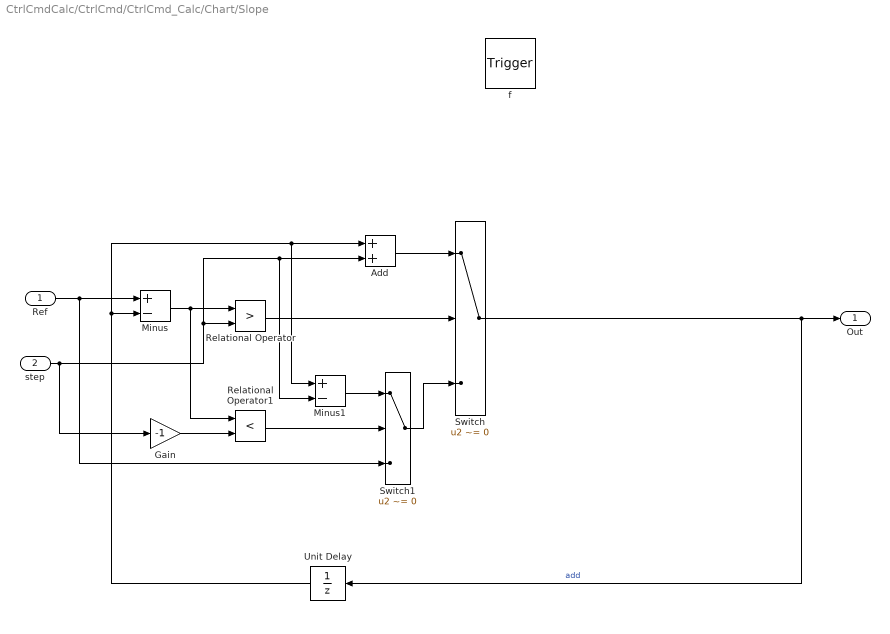
== system CtrlCmdCalc/CtrlCmd/CtrlCmd_Calc/Chart/Slope ==
  Ref : Inport  PortDimensions=1
  step : Inport  Port=2  PortDimensions=1
  f : TriggerPort  TriggerType=function-call  VariantControl=(inherit)
      settings: CopyFcn=Stateflow.SLINSF.SimulinkMan.removeBlockPreDeleteFcn  PreDeleteFcn=Stateflow.SLINSF.SimulinkMan.unsafePredeleteFcn
  Add : Sum
  Gain : Gain  Gain=-1  ParamDataTypeStr=single  OutDataTypeStr=single
  Minus : Sum  Inputs=+-  OutDataTypeStr=single
  Minus1 : Sum  Inputs=+-
  Relational Operator : RelationalOperator  Operator=>  OutDataTypeStr=boolean  RndMeth=Simplest  InputSameDT=off
  Relational Operator1 : RelationalOperator  Operator=<  OutDataTypeStr=boolean  RndMeth=Simplest  InputSameDT=off
  Switch : Switch  Criteria=u2 ~= 0  SaturateOnIntegerOverflow=off  InputSameDT=off
  Switch1 : Switch  Criteria=u2 ~= 0  SaturateOnIntegerOverflow=off  InputSameDT=off
  Unit Delay : UnitDelay  SampleTime=-1  HasFrameUpgradeWarning=on
  Out : Outport
  wires:
  Gain/1 -> Relational Operator1/2
  step/1 -> Gain/1, Minus1/2, Add/2, Relational Operator/2
  Minus/1 -> Relational Operator1/1, Relational Operator/1
  Ref/1 -> Switch1/3, Minus/1
  Switch/1 -> Unit Delay/1, Out/1  "add"
  Minus1/1 -> Switch1/1
  Relational Operator/1 -> Switch/2
  Switch1/1 -> Switch/3
  Add/1 -> Switch/1
  Relational Operator1/1 -> Switch1/2
  Unit Delay/1 -> Add/1, Minus1/1, Minus/2

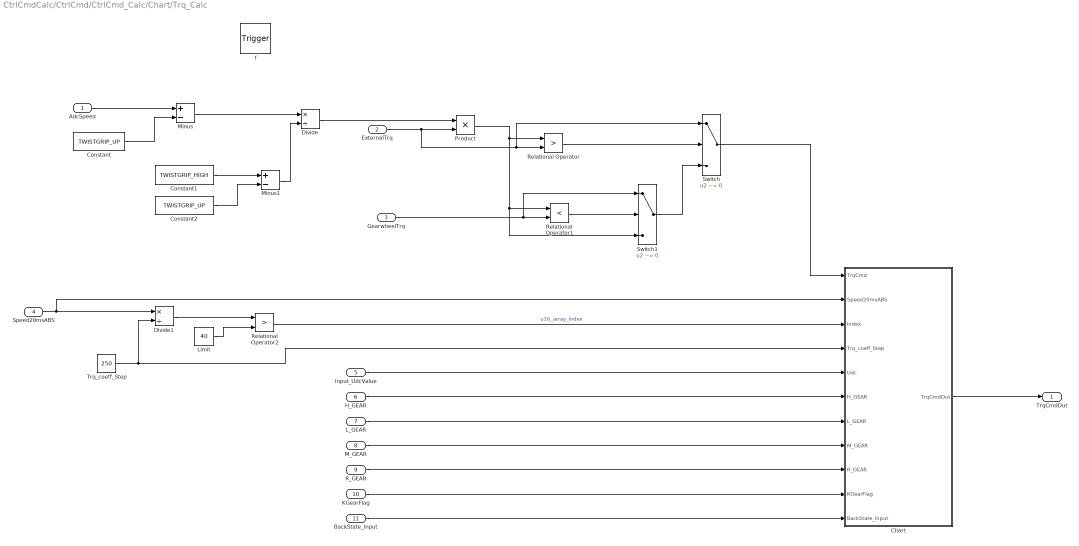
== system CtrlCmdCalc/CtrlCmd/CtrlCmd_Calc/Chart/Trq_Calc ==
  AdcSpeed : Inport
  ExternalTrq : Inport  Port=2
  GearwheelTrq : Inport  Port=3
  Speed20msABS : Inport  Port=4
  Input_UdcValue : Inport  Port=5
  H_GEAR : Inport  Port=6
  L_GEAR : Inport  Port=7
  M_GEAR : Inport  Port=8
  R_GEAR : Inport  Port=9
  KGearFlag : Inport  Port=10
  BackState_Input : Inport  Port=11
  f : TriggerPort  TriggerType=function-call  VariantControl=(inherit)
      settings: CopyFcn=Stateflow.SLINSF.SimulinkMan.removeBlockPreDeleteFcn  PreDeleteFcn=Stateflow.SLINSF.SimulinkMan.unsafePredeleteFcn
  Chart : Stateflow chart  TreatAsAtomicUnit=on
      settings: PortSchema="{\"entries\":[{\"content\":{\"sides\":[{\"content\":{\"connectorIds\":[\"In1\",\"In10\",\"In2\",\"In3\",\"In4\",\"In5\",\"In6\",\"In7\",\"In8\",\"In9\",\"In11\"]},\"type\":\"ConnectorPlacement.EquallySpacedRectSide\",\"uuid\":\"ed0f3947-753f-4d71-8a3e-ff2a2b85ce84\"},{\"content\":{\"connectorIds\":[\"Out1\"],\"side\":\"RIGHT\"},\"type\":\"ConnectorPlacement.EquallySpacedRectSide\",\"uuid\":\"e89e2f35-65d0-4132-855f-2fc9a4ff3853\"},{\"content\":{\"connectorIds\":[],\"side\":\"TOP\"},\"type\":\"ConnectorPlacement.EquallySpacedRectSide\",\"uuid\":\"c4629dfb-57bb-42cd-82c4-d7be2a8db829\"}]},\"type\":\"ConnectorPlacement.EquallySpacedConnector\",\"uuid\":\"225a5be7-8395-4bd6-b437-056ae3acac22\"}],\"packageUris\":[\"http://schema.mathworks.com/mf0/Connector/R2020b\"],\"version\":\"1.0\"}"
  Constant : Constant  Value=TWISTGRIP_UP
  Constant1 : Constant  Value=TWISTGRIP_HIGH
  Constant2 : Constant  Value=TWISTGRIP_UP
  Divide : Product  Inputs=*/
  Divide1 : Product  Inputs=*/  OutDataTypeStr=uint16
  Limit : Constant  Value=40  OutDataTypeStr=uint16
  Minus : Sum  Inputs=+-
  Minus1 : Sum  Inputs=+-
  Product : Product
  Relational Operator : RelationalOperator  Operator=>  OutDataTypeStr=boolean  RndMeth=Simplest  InputSameDT=off
  Relational Operator1 : RelationalOperator  Operator=<  OutDataTypeStr=boolean  RndMeth=Simplest  InputSameDT=off
  Relational Operator2 : RelationalOperator  Operator=>  OutDataTypeStr=boolean  RndMeth=Simplest  InputSameDT=off
  Switch : Switch  Criteria=u2 ~= 0  SaturateOnIntegerOverflow=off  InputSameDT=off
  Switch1 : Switch  Criteria=u2 ~= 0  SaturateOnIntegerOverflow=off  InputSameDT=off
  Trq_coeff_Step : Constant  Value=250  OutDataTypeStr=uint16
  TrqCmdOut : Outport
  wires:
  AdcSpeed/1 -> Minus/1
  Constant/1 -> Minus/2
  Minus/1 -> Divide/1
  Constant1/1 -> Minus1/1
  Constant2/1 -> Minus1/2
  Minus1/1 -> Divide/2
  Divide/1 -> Product/1
  ExternalTrq/1 -> Switch/1, Relational Operator/2, Product/2
  Product/1 -> Switch1/3, Relational Operator1/1, Relational Operator/1
  Relational Operator/1 -> Switch/2
  GearwheelTrq/1 -> Switch1/1, Relational Operator1/2
  Switch1/1 -> Switch/3
  Relational Operator1/1 -> Switch1/2
  Trq_coeff_Step/1 -> Chart/3(Trq_coeff_Step), Divide1/2
  Divide1/1 -> Relational Operator2/1
  Limit/1 -> Relational Operator2/2
  Relational Operator2/1 -> Chart/2(Index)  "u16_array_index"
  Input_UdcValue/1 -> Chart/4(Udc)
  H_GEAR/1 -> Chart/5(H_GEAR)
  M_GEAR/1 -> Chart/7(M_GEAR)
  R_GEAR/1 -> Chart/8(R_GEAR)
  L_GEAR/1 -> Chart/6(L_GEAR)
  KGearFlag/1 -> Chart/9(KGearFlag)
  Speed20msABS/1 -> Divide1/1, Chart/10(Speed20msABS)
  Switch/1 -> Chart/1(TrqCmd)
  BackState_Input/1 -> Chart/11(BackState_Input)
  Chart/1(TrqCmdOut) -> TrqCmdOut/1

== system CtrlCmdCalc/CtrlCmd/CtrlCmd_Calc/Chart/Vehicle_Stable ==
  SpeedIn : Inport  OutDataTypeStr=single
  SpeedLimit : Inport  Port=2  OutDataTypeStr=single  PortDimensions=1
  Torque : Inport  Port=3  OutDataTypeStr=single  PortDimensions=1
  f : TriggerPort  TriggerType=function-call  VariantControl=(inherit)
      settings: CopyFcn=Stateflow.SLINSF.SimulinkMan.removeBlockPreDeleteFcn  PreDeleteFcn=Stateflow.SLINSF.SimulinkMan.unsafePredeleteFcn
  MATLAB Function : MATLAB Function  TreatAsAtomicUnit=on
  Flag : Outport
  wires:
  SpeedLimit/1 -> MATLAB Function/2(SpeedLimit)
  SpeedIn/1 -> MATLAB Function/1(Speed)
  Torque/1 -> MATLAB Function/3(TorqueFdk)
  MATLAB Function/1(Vehicle_Stable_Flag) -> Flag/1

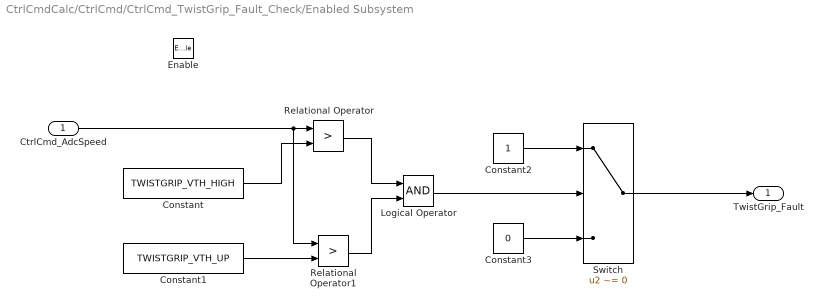
== system CtrlCmdCalc/CtrlCmd/CtrlCmd_TwistGrip_Fault_Check/Enabled Subsystem ==
  CtrlCmd_AdcSpeed : Inport
  Enable : EnablePort
  Constant : Constant  Value=TWISTGRIP_VTH_HIGH
  Constant1 : Constant  Value=TWISTGRIP_VTH_UP
  Constant2 : Constant  OutDataTypeStr=uint8
  Constant3 : Constant  Value=0  OutDataTypeStr=uint8
  Logical Operator : Logic  AllPortsSameDT=off  OutDataTypeStr=boolean
  Relational Operator : RelationalOperator  Operator=>  OutDataTypeStr=boolean  RndMeth=Simplest  InputSameDT=off
  Relational Operator1 : RelationalOperator  Operator=>  OutDataTypeStr=boolean  RndMeth=Simplest  InputSameDT=off
  Switch : Switch  Criteria=u2 ~= 0  SaturateOnIntegerOverflow=off  InputSameDT=off
  TwistGrip_Fault : Outport
  wires:
  CtrlCmd_AdcSpeed/1 -> Relational Operator1/1, Relational Operator/1
  Constant/1 -> Relational Operator/2
  Constant1/1 -> Relational Operator1/2
  Relational Operator/1 -> Logical Operator/1
  Relational Operator1/1 -> Logical Operator/2
  Constant2/1 -> Switch/1
  Constant3/1 -> Switch/3
  Logical Operator/1 -> Switch/2
  Switch/1 -> TwistGrip_Fault/1

== stateflow chart CtrlCmdCalc/CtrlCmd/CtrlCmd_Mode_Seclect/Chart1 ==
  (default) -> (junction 7)
  (junction 7) -> (junction 9) [order 1] : [SelfCheckOverFlag == 0 || PreChargeOverFlag == 0]
  (junction 7) -> (junction 14) [order 2]
  (junction 9) -> (junction 11) : {
      | WorkCmdAnalogRunCmd = 0;
      | WorkCmdAnalogModeCmd = cNoneMode;
      | WorkCmdAnalogTorqueCmd = 0;
      | }
  (junction 11) -> (junction 54)
  (junction 14) -> (junction 29) [order 1]
  (junction 29) -> (junction 19) [order 1] : [HighSpeedZeroTrqFlag == 0 && abs(TorqueCtrl_TorqueCmdFilter)<1&&abs(AnalogTorqueCmdDelay)<1&&TGFlagDelay == false]
  (junction 14) -> (junction 51) [order 2]
  (junction 29) -> (junction 31) [order 2] : {
      | TimeCnt=0;
      | StanByFlag=false;
      | }
  (junction 19) -> (junction 22) : {
      | TimeCnt = TimeCnt +1
      | }
  (junction 22) -> (junction 25) [order 1] : [TimeCnt>=500]{TimeCnt=500;StanByFlag=true}
  (junction 22) -> (junction 25) [order 2]
  (junction 25) -> (junction 33)
  (junction 33) -> (junction 31)
  (junction 31) -> (junction 36)
  (junction 36) -> (junction 51)
  (junction 54) -> (junction 36)
  (junction 51) -> (junction 49)
  data: SelfCheckOverFlag input; PreChargeOverFlag input; WorkCmdAnalogRunCmd output uint16 =0; WorkCmdAnalogModeCmd output uint16; cNoneMode parameter; WorkCmdAnalogTorqueCmd output single =0; HighSpeedZeroTrqFlag input; TorqueCtrl_TorqueCmdFilter input; TGFlagDelay input; AnalogTorqueCmdDelay input; TimeCnt local uint16 =0; StanByFlag local uint8 =0

== stateflow chart CtrlCmdCalc/CtrlCmd/CtrlCmd_Calc/Chart ==
  state Flag = Vehicle_Stable(SpeedIn,SpeedLimit,Torque) [function]
  state TrqCmdOut = Trq_Calc(AdcSpeed,ExternalTrq,GearwheelTrq,Speed20msABS,Input_UdcValue,H_GEAR,L_GEAR,M_GEAR,R_GEAR,KGearFlag,BackState_Input) [function]
  state Out = Slope(Ref,step) [function]
  (default) -> (junction 5)
  (junction 5) -> (junction 7) [order 1] : [WorkStateBefore == POWER_ON && WorkState == STANDBY && PInitState==0]
  (junction 5) -> (junction 19) [order 2]
  (junction 7) -> (junction 13) [order 2]
  (junction 7) -> (junction 13) [order 1] : [Speed20msAbs>20]{KGearFlag=H_GEAR}
  (junction 13) -> (junction 19) : {PInitState=1}
  (junction 19) -> (junction 21) [order 2]
  (junction 19) -> (junction 21) [order 1] : [T_Cnt>=PTIME]{T_Cnt=0}
  (junction 21) -> (junction 27)
  (junction 27) -> (junction 29) [order 1] : [KGearFlag==P_GEAR && SelfCheckOverFlag==1]
  (junction 27) -> (junction 33) [order 2]
  (junction 29) -> (junction 37) [order 2]
  (junction 29) -> (junction 37) [order 1] : [Brake_State_Old==false && BrakeState_Input==true]{Brake_In_Flag=true}
  (junction 37) -> (junction 42) [order 2]
  (junction 37) -> (junction 42) [order 1] : [Brake_In_Flag==true && BrakeState_Input==false]
      | {KGearFlag=M_GEAR;Brake_In_Flag=false;T_Cnt=0}
  (junction 42) -> (junction 33)
  (junction 33) -> (junction 46) : {Brake_State_Old = BrakeState_Input}
  (junction 46) -> (junction 50) [order 1] : [AdcSpeed>TWISTGRIP_UP]
  (junction 46) -> (junction 75) [order 2]
  (junction 50) -> (junction 55) : {T_Cnt=0;TGFlag=true}
  (junction 55) -> (junction 53)
  (junction 53) -> (junction 60) [order 1] : [KGearFlag !=P_GEAR]
  (junction 60) -> (junction 62) [order 2]
  (junction 53) -> (junction 65) [order 2] : {AdcSpeed=0}
  (junction 60) -> (junction 62) [order 1] : [BrakeState_Input ==0]{AdcSpeed=0}
  (junction 62) -> (junction 65)
  (junction 65) -> (junction 99)
  (junction 75) -> (junction 68) [order 1] : {TGFlag = false}
  (junction 68) -> (junction 70) [order 1] : [BrakeState_Input==0]{T_Cnt=0}
  (junction 68) -> (junction 70) [order 2] : {T_Cnt = T_Cnt+1}
  (junction 75) -> (junction 96) [order 2]
  (junction 70) -> (junction 58) : {StableFlag = Vehicle_Stable(500,Speed20msAbs,TorqueFeedback)}
  (junction 58) -> (junction 73) [order 1] : [StableFlag==1]
  (junction 73) -> (junction 90) [order 2] : {KGearFlag = R_GEAR}
  (junction 58) -> (junction 85) [order 2]
  (junction 73) -> (junction 90) [order 1] : [BackState_Input==0&&KGearFlag!=P_GEAR]{KGearFlag = R_GEAR}
  (junction 90) -> (junction 87) : {AntiTheftFlag = AntiTheftState_Input}
  (junction 85) -> (junction 96)
  (junction 87) -> (junction 85)
  (junction 96) -> (junction 101)
  (junction 99) -> (junction 101)
  (junction 101) -> (junction 104)
  (junction 104) -> (junction 112) [order 1] : [TwistGrip_Fault==true || UdcUnderFault==true || UdcOverFault==true || TZFault==true || TwistGrip_Warn==true]
  (junction 104) -> (junction 114) [order 2]
  (junction 112) -> (junction 116) : {
      | AdcSpeed=0;
      | TorqueCmd=0;
      | Time_cnt=0;
      | }
  (junction 114) -> (junction 120) [order 1] : [TGFlag==true]
  (junction 114) -> (junction 149) [order 2]
  (junction 120) -> (junction 140) : {
      | Gearwheel_TrqAdd=0;
      | TorqueCmd = Trq_Calc(AdcSpeed,ExternalTorque,Gearwheel_TrqAdd,Speed20msAbs,UdcValue,H_GEAR,L_GEAR,M_GEAR,R_GEAR,KGearFlag,BackState_Input)
      | Time_cnt=0;
      | }
  (junction 116) -> (junction 257)
  (junction 140) -> (junction 254)
  (junction 149) -> (junction 166) [order 1] : {
      | Time_cnt = Time_cnt+1;
      | Trq_External_Max=ExternalTorque
      | }
  (junction 166) -> (junction 169) [order 1] : [Trq_External_Max>ParamCfg_MaxTorque_u16*0.1]
      | {Trq_External_Max=ParamCfg_MaxTorque_u16*0.1}
  (junction 169) -> (junction 173) : {Gearwheel_TrqAdd=Trq_External_Max * 0.035}
  (junction 173) -> (junction 175) [order 1] : [Gearwheel_TrqAdd<0.3]{Gearwheel_TrqAdd=0.3}
  (junction 173) -> (junction 175) [order 2]
  (junction 166) -> (junction 169) [order 2]
  (junction 175) -> (junction 178) [order 2]
  (junction 149) -> (junction 260) [order 2]
  (junction 175) -> (junction 178) [order 1] : [Gearwheel_TrqAdd>0.7]{Gearwheel_TrqAdd=0/7}
  (junction 178) -> (junction 181) [order 2]
  (junction 178) -> (junction 181) [order 1] : [Speed20msAbs<100]{Gearwheel_TrqAdd=0.05}
  (junction 181) -> (junction 184)
  (junction 184) -> (junction 186) [order 1] : {Time_cnt>=80}
  (junction 184) -> (junction 188) [order 2]
  (junction 186) -> (junction 188) : {
      | Time_cnt=80;
      | Gearwheel_TrqAdd=Gearwheel_TrqAdd*0.1
      | }
  (junction 188) -> (junction 191) : {Gearwheel_TrqAdd=0}
  (junction 191) -> (junction 193)
  (junction 193) -> (junction 195) [order 1] : [KGearFlag==P_GEAR]
  (junction 193) -> (junction 197) [order 2]
  (junction 195) -> (junction 216) : {TorqueCmd=Slope(0,1)}
  (junction 216) -> (junction 249)
  (junction 197) -> (junction 218) [order 1] : {Nothing=1}
  (junction 218) -> (junction 221) [order 2] : [KGearFlag == R_GEAR]
  (junction 197) -> (junction 246) [order 2]
  (junction 218) -> (junction 235) [order 1]
  (junction 221) -> (junction 223) : {Nothing=2}
  (junction 223) -> (junction 225) [order 1] : [Speed20ms<-100]{TorqueCmd = Slope(0,1)}
  (junction 223) -> (junction 225) [order 2] : {TorqueCmd = Slope(Gearwheel_TrqAdd,1)}
  (junction 225) -> (junction 229)
  (junction 235) -> (junction 234) [order 1] : {Nothing=3}
  (junction 234) -> (junction 237) [order 2] : {TorqueCmd = Slope(0-Gearwheel_TrqAdd,1)}
  (junction 235) -> (junction 240) [order 2]
  (junction 234) -> (junction 237) [order 1] : [Speed20ms>100]{TorqueCmd = Slope(0,1)}
  (junction 237) -> (junction 240)
  (junction 240) -> (junction 231)
  (junction 229) -> (junction 231)
  (junction 231) -> (junction 244)
  (junction 246) -> (junction 260) [order 2]
  (junction 244) -> (junction 246)
  (junction 249) -> (junction 244)
  (junction 260) -> (junction 263)
  (junction 246) -> (junction 252) [order 1]
  (junction 254) -> (junction 252)
  (junction 257) -> (junction 254)
  (junction 263) -> (junction 265) [order 1] : [UdcUnderFault==true || UdcOverFault==true]
  (junction 263) -> (junction 270) [order 2]
  (junction 265) -> (junction 267) : {Fault_Stay_Flag=1}
  (junction 270) -> (junction 272) [order 1] : [TGFlag==0]
  (junction 270) -> (junction 281) [order 2]
  (junction 272) -> (junction 276) : {Fault_Stay_Flag=0}
  (junction 276) -> (junction 281)
  (junction 267) -> (junction 276)
  (junction 281) -> (junction 283) [order 2]
  (junction 281) -> (junction 283) [order 1] : [Fault_Stay_Flag==1]{TorqueCmd=0}
  (junction 283) -> (junction 288)
  data: SpeedIn function_input single; SpeedLimit function_input single size=1; Torque function_input single size=1; Flag function_output; AdcSpeed function_input; ExternalTrq function_input; GearwheelTrq function_input; Speed20msABS function_input; Input_UdcValue function_input; H_GEAR function_input; L_GEAR function_input; M_GEAR function_input; R_GEAR function_input; KGearFlag function_input; BackState_Input function_input; TrqCmdOut function_output; Ref function_input size=1; step function_input size=1; Out function_output; UdcValue input; TwistGrip_Fault input; TwistGrip_Warn input; UdcUnderFault input; UdcOverFault input; TZFault input; AntiTheftState_Input input; TGFlag output uint16 =0; BrakeState_Input input; WorkStateBefore input; WorkState input; ExternalTorque input; TorqueFeedback input; POWER_ON parameter; STANDBY parameter; PInitState local uint8 =0; Speed20msAbs input; KGearFlag output uint16 =0; H_GEAR input; T_Cnt local uint16 =0; PTIME parameter; SelfCheckOverFlag input; P_GEAR input; Brake_In_Flag local uint8 =0; Brake_State_Old local uint8 =0; M_GEAR input; TWISTGRIP_UP parameter; AdcSpeed data_store_memory; StableFlag local uint16 =0; R_GEAR input; AntiTheftFlag output uint16 =0; TorqueCmd output single; Time_cnt local uint16 =0; Gearwheel_TrqAdd output single =0; L_GEAR input; BackState_Input input; Trq_External_Max local single; ParamCfg_MaxTorque_u16 parameter; Nothing local uint8 =1; Speed20ms input; Fault_Stay_Flag local uint8 =0

== stateflow chart CtrlCmdCalc/CtrlCmd/CtrlCmd_Mode_Seclect/Chart ==
  (default) -> (junction 7)
  (junction 7) -> (junction 9) [order 1] : [SelfCheckOverFlag == 0 || PreChargeOverFlag == 0]
  (junction 7) -> (junction 90) [order 2]
  (junction 9) -> (junction 11) : {
      | WorkCmdAnalogRunCmd = 0;
      | WorkCmdAnalogModeCmd = cNoneMode;
      | WorkCmdAnalogTorqueCmd = 0;
      | }
  (junction 90) -> (junction 29) [order 1] : {m=0}
  (junction 29) -> (junction 19) [order 1] : [HighSpeedZeroTrqFlag == 0 && abs(TorqueCtrl_TorqueCmdFilter)<1&&abs(AnalogTorqueCmdDelay)<1&&TGFlagDelay == false]
  (junction 90) -> (junction 95) [order 2]
  (junction 29) -> (junction 31) [order 2] : {
      | TimeCnt=0;
      | StanByFlag=false;
      | }
  (junction 19) -> (junction 22) : {
      | TimeCnt = TimeCnt +1
      | }
  (junction 22) -> (junction 25) [order 1] : [TimeCnt>=500]{TimeCnt=500;StanByFlag=true}
  (junction 22) -> (junction 25) [order 2]
  (junction 25) -> (junction 33)
  (junction 33) -> (junction 31)
  (junction 31) -> (junction 77)
  (junction 77) -> (junction 98) [order 1] : [StanByFlag == 1 || KGearFlagDelay == PGEAR]
  (junction 77) -> (junction 100) [order 2] : {
      | WorkCmdAnalogRunCmd = 1;
      | WorkCmdAnalogModeCmd=cTorqueLoopMode;
      | WorkCmdAnalogTorqueCmd
      | }
  (junction 98) -> (junction 106) : {
      | WorkCmdAnalogRunCmd=0;
      | WorkCmdAnalogModeCmd=cNoneMode;
      | WorkCmdAnalogTorqueCmd = 0;
      | }
  (junction 106) -> (junction 100)
  (junction 100) -> (junction 110)
  (junction 110) -> (junction 112) [order 1] : [Speed20msAbs >1000]{WorkCmdAnalogRunCmd=1}
  (junction 110) -> (junction 112) [order 2]
  (junction 112) -> (junction 116)
  (junction 116) -> (junction 95)
  (junction 95) -> (junction 119)
  (junction 11) -> (junction 119)
  (junction 119) -> (junction 122)
  data: SelfCheckOverFlag input; PreChargeOverFlag input; WorkCmdAnalogRunCmd output uint16 =0; WorkCmdAnalogModeCmd output uint16; cNoneMode parameter; WorkCmdAnalogTorqueCmd output single =0; HighSpeedZeroTrqFlag input; TorqueCtrl_TorqueCmdFilter input; TGFlagDelay input; AnalogTorqueCmdDelay input; TorqueCmdDelay input; Speed20msAbs input; TimeCnt local uint16 =0; StanByFlag local uint8 =0; m output uint8 =0; KGearFlagDelay input; PGEAR input; cTorqueLoopMode parameter

== matlab function CtrlCmdCalc/CtrlCmd/CtrlCmd_Calc/Chart/Vehicle_Stable/MATLAB Function ==
  data: Speed input; Vehicle_Stable_Flag output; SpeedLimit input; TorqueFdk input
function Vehicle_Stable_Flag = CtrlCmd_Vehicle_Stable(Speed, SpeedLimit, TorqueFdk)
% CtrlCmd_Vehicle_Stable 判断车辆是否处于静止稳定状态
% 输入参数:
%   Speed         - 速度判定阈值(单位与SpeedLimit一致)
%   SpeedLimit    - 实际测量的车辆速度(20ms周期更新的ABS速度)
%   TorqueFdk     - 实际扭矩反馈值
% 输出参数:
%   Vehicle_Stable_Flag - 车辆稳定标志(uint16类型: 1=稳定静止, 0=不稳定)
% 说明:
%   该函数需以20ms固定周期调用，连续6个周期(120ms)同时满足条件才判定为稳定

    % 声明持久变量(内部状态，函数调用间保持值不变)
    persistent VehStable_Count Internal_Stable_Flag
    
    % 持久变量初始化(仅在程序第一次调用该函数时执行一次)
    if isempty(VehStable_Count)
        VehStable_Count = uint16(0);
        Internal_Stable_Flag = uint16(0);
    end

    % 核心判断逻辑：速度低于阈值 且 扭矩接近0
    if (SpeedLimit < Speed) && (abs(TorqueFdk) < 1.0)
        % 只有当尚未判定为稳定时才进行计数
        if (Internal_Stable_Flag == 0)
            VehStable_Count = VehStable_Count + 1;
            % 连续6个周期满足条件则判定为稳定
            if (VehStable_Count > 5)
                VehStable_Count = uint16(0);
                Internal_Stable_Flag = uint16(1);
            end
        end
    else
        % 任一条件不满足则重置计数器和稳定标志
        VehStable_Count = uint16(0);
        Internal_Stable_Flag = uint16(0);
    end

    % 将内部状态赋值给输出参数
    Vehicle_Stable_Flag = Internal_Stable_Flag;
end

== stateflow chart CtrlCmdCalc/CtrlCmd/CtrlCmd_Calc/Chart/Trq_Calc/Chart ==
  note: Do not put any code along
      | the transitions that run
      | down the right side!
  (default) -> (junction 53)
  (junction 28) -> (junction 29) [order 1] : [KGearFlag == R_GEAR]
  (junction 54) -> (junction 28)
  (junction 53) -> (junction 54) [order 1] : [Udc>67]
  (junction 28) -> (junction 32) [order 2]
  (junction 29) -> (junction 30) : {
      | TrqFront = Trq_coeff_Arr_Back_72V[Index] *0.01
      | TrqBehind = Trq_coeff_Arr_Back_72V[Index+1] *0.01
      | }
  (junction 53) -> (junction 94) [order 2]
  (junction 30) -> (junction 31)
  (junction 31) -> (junction 35)
  (junction 32) -> (junction 33) [order 1] : [KGearFlag == L_GEAR ]
  (junction 32) -> (junction 36) [order 2]
  (junction 33) -> (junction 34) : {
      | TrqFront = Trq_coeff_Arr_HSP_72V[Index] *0.01
      | TrqBehind = Trq_coeff_Arr_HSP_72V[Index+1] *0.01
      | }
  (junction 34) -> (junction 35)
  (junction 35) -> (junction 39)
  (junction 36) -> (junction 37) [order 1] : [KGearFlag == M_GEAR]
  (junction 36) -> (junction 40) [order 2]
  (junction 37) -> (junction 38) : {
      | TrqFront = Trq_coeff_Arr_HSP_72V[Index] *0.01
      | TrqBehind = Trq_coeff_Arr_HSP_72V[Index+1] *0.01
      | }
  (junction 94) -> (junction 96) [order 1] : [KGearFlag == R_GEAR]
  (junction 96) -> (junction 95) : {
      | TrqFront = Trq_coeff_Arr_Back_60V[Index] *0.01
      | TrqBehind = Trq_coeff_Arr_Back_60V[Index+1] *0.01
      | }
  (junction 94) -> (junction 99) [order 2]
  (junction 38) -> (junction 39)
  (junction 39) -> (junction 43)
  (junction 40) -> (junction 41) [order 1] : [KGearFlag == H_GEAR]
  (junction 95) -> (junction 93)
  (junction 40) -> (junction 44) [order 2] : {
      | TrqFront = Trq_coeff_Arr_HSP_72V[Index] *0.01
      | TrqBehind = Trq_coeff_Arr_HSP_72V[Index+1] *0.01
      | }
  (junction 41) -> (junction 42) : {
      | TrqFront = Trq_coeff_Arr_HSP_72V[Index] *0.01
      | TrqBehind = Trq_coeff_Arr_HSP_72V[Index+1] *0.01
      | }
  (junction 93) -> (junction 100)
  (junction 99) -> (junction 97) [order 1] : [KGearFlag == L_GEAR ]
  (junction 97) -> (junction 98) : {
      | TrqFront = Trq_coeff_Arr_HSP_60V[Index] *0.01
      | TrqBehind = Trq_coeff_Arr_HSP_60V[Index+1] *0.01
      | }
  (junction 99) -> (junction 101) [order 2]
  (junction 42) -> (junction 43)
  (junction 43) -> (junction 45)
  (junction 98) -> (junction 100)
  (junction 100) -> (junction 103)
  (junction 45) -> (junction 44)
  (junction 101) -> (junction 104) [order 1] : [KGearFlag == M_GEAR]
  (junction 44) -> (junction 46)
  (junction 104) -> (junction 102) : {
      | TrqFront = Trq_coeff_Arr_HSP_60V[Index] *0.01
      | TrqBehind = Trq_coeff_Arr_HSP_60V[Index+1] *0.01
      | }
  (junction 101) -> (junction 105) [order 2]
  (junction 102) -> (junction 103)
  (junction 103) -> (junction 108)
  (junction 105) -> (junction 111) [order 1] : [KGearFlag == H_GEAR]
  (junction 111) -> (junction 106) : {
      | TrqFront = Trq_coeff_Arr_HSP_60V[Index] *0.01
      | TrqBehind = Trq_coeff_Arr_HSP_60V[Index+1] *0.01
      | }
  (junction 105) -> (junction 109) [order 2] : {
      | TrqFront = Trq_coeff_Arr_HSP_60V[Index] *0.01
      | TrqBehind = Trq_coeff_Arr_HSP_60V[Index+1] *0.01
      | }
  (junction 106) -> (junction 108)
  (junction 108) -> (junction 110)
  (junction 110) -> (junction 109)
  (junction 109) -> (junction 107)
  (junction 46) -> (junction 107)
  (junction 107) -> (junction 113) [order 2]
  (junction 107) -> (junction 113) [order 1] : [TrqFront<0]{TrqFront=0}
  (junction 113) -> (junction 117) [order 2]
  (junction 113) -> (junction 117) [order 1] : [TrqBehind<0]{TrqBehind=0}
  (junction 117) -> (junction 120) : {Trq_limit_coeff = TrqFront - (((TrqFront - TrqBehind) * (Speed20msABS - ((Trq_coeff_Step)*Index))) / ((Trq_coeff_Step)));}
  (junction 120) -> (junction 126) : {TrqCmdOut = TrqCmd*Trq_limit_coeff}
  (junction 126) -> (junction 129)
  (junction 129) -> (junction 131) [order 1] : [KGearFlag==R_GEAR && BackState_Input==0]
  (junction 129) -> (junction 136) [order 2]
  (junction 131) -> (junction 134) : {TrqCmdOut = TrqCmdOut*-1}
  (junction 136) -> (junction 138) [order 1] : [(KGearFlag!=R_GEAR && BackState_Input==0) || ((R_GEAR == KGearFlag) && (1 == BackState_Input))]
  (junction 136) -> (junction 142) [order 2] : {TrqCmdOut = TrqCmdOut}
  (junction 138) -> (junction 140) : {TrqCmdOut=0}
  (junction 140) -> (junction 142)
  (junction 134) -> (junction 140)
  (junction 142) -> (junction 147) [order 2] : {TrqCmdOut = -1*TrqCmdOut}
  (junction 142) -> (junction 147) [order 1] : [MOTORDIR]{TrqCmdOut = TrqCmdOut}
  (junction 147) -> (junction 151)
  data: TrqCmd input; Index input; Trq_coeff_Step input; Udc input; H_GEAR input; L_GEAR input; M_GEAR input; R_GEAR input; KGearFlag input; Trq_coeff_Arr_Back_72V parameter; TrqBehind local single =0; TrqFront local single =0; Trq_coeff_Arr_HSP_60V parameter; Trq_coeff_Arr_HSP_72V parameter; Trq_coeff_Arr_Back_60V parameter; Trq_limit_coeff local single =0; Speed20msABS input; TrqCmdOut output single =0; BackState_Input input; MOTORDIR parameter
